simulink model "Progetto_drone_2"  (R2024b)
settings: Solver=VariableStepAuto  StartTime=0.0  StopTime=20  RelTol=1e-3
settings Model: Creator=sugam  LastModifiedBy=3204480343

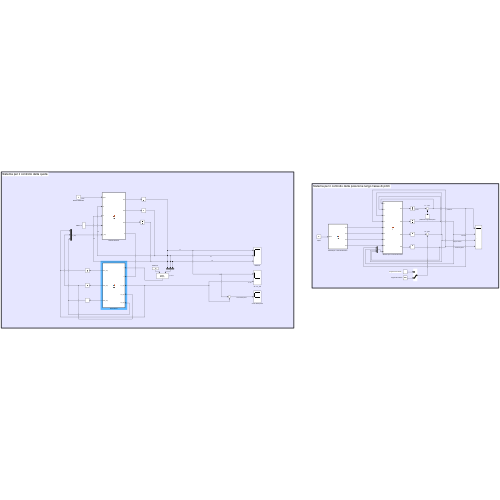
[thumbnail: Simulink's stored preview of the top-level diagram]
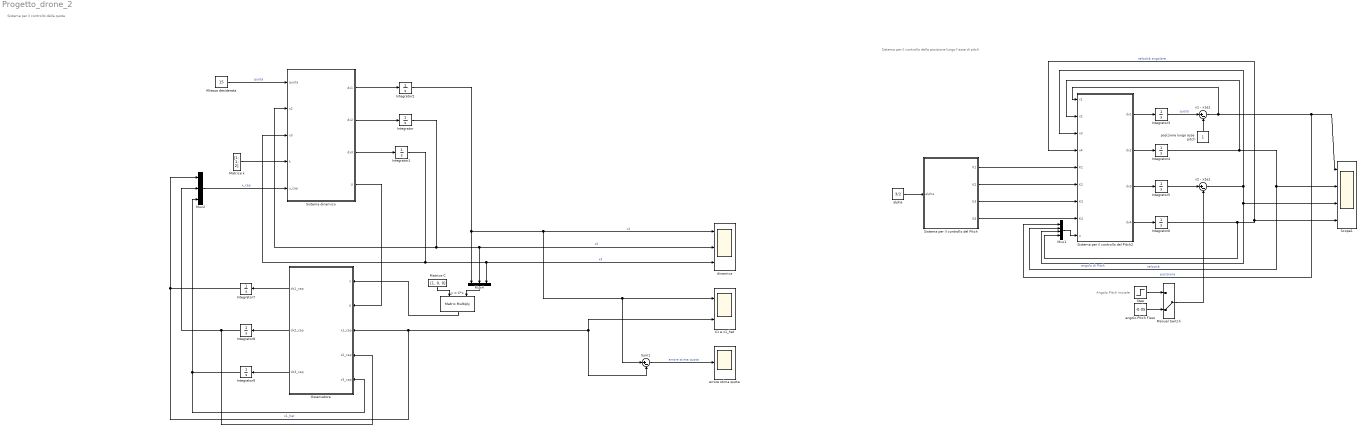
== system Progetto_drone_2 ==
  note: Angolo Pitch iniziale
  note: Sistema per il controllo della quota
  note: Sistema per il controllo della posizione lungo l'asse di pitch
  Altezza desiderata : Constant  Value=15
  Integrator{,1..6} (7 alike) : Integrator
  Integrator7 : Integrator  InitialCondition=2
  Integrator8 : Integrator  InitialCondition=2
  Integrator9 : Integrator  InitialCondition=2
  Manual Switch : ManualSwitch  CurrentSetting=0
  Matrice C : Constant  Value=[1, 0, 0]  VectorParams1D=off
  Matrice k : Constant  Value=[1; 1; 2]  VectorParams1D=off
  Mux1 : Mux
  Mux2 : Mux  Inputs=3
  Mux4 : Mux  Inputs=3
  Osservatore : MATLAB Function  TreatAsAtomicUnit=on
  Scope1 : Scope  NumInputPorts=4
  Sistema dinamico : MATLAB Function  TreatAsAtomicUnit=on
  Sistema per il controllo del Pitch : MATLAB Function  TreatAsAtomicUnit=on
  Sistema per il controllo del Pitch2 : MATLAB Function  TreatAsAtomicUnit=on
  Step : Step  Time=0.01  Before=0.05  After=0  SampleTime=0
  Sum1 : Sum  Inputs=|+-
  X1 e x1_hat : Scope  NumInputPorts=2
  alpha : Constant  Value=3/2
  angolo Pitch Fisso : Constant  Value=-0.05
  dinamica : Scope  NumInputPorts=3
  errore stima quota : Scope
  posizione lungo asse pitch : Constant
  x1 - x1e1 : Sum  Inputs=|+-
  x2 - x2e1 : Sum  Inputs=|+-
  y = C*x : Product  Multiplication=Matrix(*)
  wires:
  alpha/1 -> Sistema per il controllo del Pitch/1(alpha)
  Sistema per il controllo del Pitch/1(K1) -> Sistema per il controllo del Pitch2/5(K1)
  Sistema per il controllo del Pitch/2(K2) -> Sistema per il controllo del Pitch2/6(K2)
  Sistema per il controllo del Pitch/3(K3) -> Sistema per il controllo del Pitch2/7(K3)
  Sistema per il controllo del Pitch/4(K4) -> Sistema per il controllo del Pitch2/8(K4)
  Sistema per il controllo del Pitch2/1(dx1) -> Integrator3/1
  Sistema per il controllo del Pitch2/2(dx2) -> Integrator4/1
  Sistema per il controllo del Pitch2/3(dx3) -> Integrator5/1
  Sistema per il controllo del Pitch2/4(dx4) -> Integrator6/1
  Integrator4/1 -> Sistema per il controllo del Pitch2/2(x2), Scope1/2, Mux1/2  "velocità"
  Integrator6/1 -> Mux1/4, Sistema per il controllo del Pitch2/4(x4), Scope1/4  "velocità angolare"
  Mux1/1 -> Sistema per il controllo del Pitch2/9(u)
  Integrator5/1 -> x2 - x2e1/1
  x2 - x2e1/1 -> Mux1/3, Scope1/3, Sistema per il controllo del Pitch2/3(x3)  "angolo di Pitch"
  Step/1 -> Manual Switch/1
  angolo Pitch Fisso/1 -> Manual Switch/2
  Manual Switch/1 -> x2 - x2e1/2
  posizione lungo asse pitch/1 -> x1 - x1e1/2
  Integrator3/1 -> x1 - x1e1/1  "quota"
  x1 - x1e1/1 -> Sistema per il controllo del Pitch2/1(x1), Mux1/1, Scope1/1  "posizione"
  y = C*x/1 -> Osservatore/1(y)
  Matrice C/1 -> y = C*x/1
  Matrice k/1 -> Sistema dinamico/4(k)
  Mux4/1 -> y = C*x/2
  Mux2/1 -> Sistema dinamico/5(x_cap)  "x_cap"
  Osservatore/2(dx2_cap) -> Integrator8/1
  Osservatore/1(dx1_cap) -> Integrator7/1
  Osservatore/3(dx3_cap) -> Integrator9/1
  Sistema dinamico/3(dx3) -> Integrator1/1
  Integrator7/1 -> X1 e x1_hat/2, Sum1/2, Osservatore/3(x1_cap), Mux2/1  "x1_hat"
  Integrator/1 -> Mux4/2, dinamica/2, Sistema dinamico/2(x2)  "x2"
  Sistema dinamico/1(dx1) -> Integrator2/1
  Sum1/1 -> errore stima quota/1  "errore stima quota"
  Integrator2/1 -> Mux4/1, Sum1/1, X1 e x1_hat/1, dinamica/1  "x1"
  Integrator8/1 -> Osservatore/4(x2_cap), Mux2/2
  Sistema dinamico/2(dx2) -> Integrator/1
  Altezza desiderata/1 -> Sistema dinamico/1(quota)  "quota"
  Integrator1/1 -> Mux4/3, dinamica/3, Sistema dinamico/3(x3)  "x3"
  Integrator9/1 -> Mux2/3, Osservatore/5(x3_cap)
  Sistema dinamico/4(U) -> Osservatore/2(U)

== matlab function Progetto_drone_2/Sistema per il controllo del Pitch2 ==
  data: x1 input; x2 input; x3 input; x4 input; K1 input; K2 input; K3 input; K4 input; u input; dx1 output; dx2 output; dx3 output; dx4 output
function [dx1, dx2, dx3, dx4] = fcn(x1, x2, x3, x4, K1, K2, K3, K4, u)
%Inizializzazione dei parametri inerenti il drone e l'ambiente
g = 9.81;           %forza di gravità che agisce sul drone
I = (1/10)*eye(1);         % momento di inerzia -> valore consiglito 0.02 Kg*m^2
P = 1;              % P parametro che converte l'ingresso 'u' in una coppia per i motori -> valore consigliato 3*10^-7 N*m*s^2

%Sistema non lineare per il controllo della quota verticale descritto dalle
%seguenti equazioni differenziali
%dx1 = x2;
%dx2 = (1/m)*(-Tsin(x3) -cx2);
%dx3 = x4;
%dx4 = (P/I)*u2;

%utilizzo un controllo u1 per mantenere il drone su una quota fissa
%u1 = (T/(cos(theta))*m*g ;

%Il controllo che mi permette di stabilizzare il sistema viene calcolato
%tramite backstepping della madonna, 8 pagine de calcoli mortacci tua
u = (I/P)*(K1*u(1) + K2*u(2) + K3*u(3) + K4*u(4));

%Da questo ottengo il sistema linearizzato nell'intorno del punto di
%equilibrio (xe,ue), dove tutti gli elementi sono pari a zero tranne la x1
%che è libera
dx1 = x2;
dx2 = -g*x3;
dx3 = x4;
dx4 = (P/I)*u;

%x1 posizione lungo l'asse del pitch
%x2 velocita longitudinale
%x3 angolo di pitch
%x4 velocita angolare

== matlab function Progetto_drone_2/Sistema dinamico ==
  data: quota input; dx1 output; dx2 output; x2 input; x3 input; k input; dx3 output; x_cap input; U output
function [dx1, dx2, dx3, U] = fcn(quota, x2, x3, k, x_cap)
%Inizializzazione dei parametri inerenti il drone e l'ambiente
g = 9.81;           % forza di gravità che agisce sul drone
tau = 0.1;          % costante di tempo per generare ritardo nel controllo
ka = 0.1;           % coefficiente di proporzionalità tra x3 ed F
m = 1;              % massa del drone

x3e = sqrt(g*m/ka); % circa uguale a 9.9, x3 equlibrio 

ue = x3e;

%Il controllo che mi permette di stabilizzare il sistema viene calcolato
%tramite la legge di feedback dello stato u = -kx
U = -k(1)*(x_cap(1) - quota) - k(2)*x_cap(2) - k(3)*(x_cap(3) - sqrt(g*m/ka)) + ue ; % u_tilde = u - ue

%Sistema non lineare per il controllo della quota verticale descritto dalle
%seguenti equazioni differenziali
dx1 = x2;
dx2 = (ka/m)*x3^2 - g;
dx3 = (U - x3)/tau;

% x1 quota
% x2 velocità 
% x3 cinematica motore (spinta motore)

== matlab function Progetto_drone_2/Sistema per il controllo del Pitch ==
  data: alpha input; K1 output; K2 output; K3 output; K4 output
function [K1, K2, K3, K4] = fcn(alpha)
%inizializzazione parametri
g = 9.81;

%calcolo delle varie K che fanno parte del controllo come
%u = (I/P)*(K1*x1 + K2*x2 + K3*x3 + K4*x4)
K1 = -(2*(alpha^4) + (6*(alpha^3)) + (-4*(alpha^2)) + (-16*alpha) + (-alpha*(g^2)) -8)/g;
K2 = -(-4*alpha + (-alpha*(g^2)) -4 - (g^2))/g;
K3 = -(3*alpha + 5 + g^2);
K4 = - (3+alpha) ;

== matlab function Progetto_drone_2/Osservatore ==
  data: y input; U input; x1_cap input; x2_cap input; x3_cap input; dx1_cap output; dx2_cap output; dx3_cap output
function [dx1_cap, dx2_cap, dx3_cap] = fcn(y, U, x1_cap, x2_cap, x3_cap)
%Inizializzazione dei parametri inerenti il drone e l'ambiente
g = 9.81;           % forza di gravità che agisce sul drone
tau = 0.1;          % costante di tempo per generare ritardo nel controllo
ka = 0.1;           % coefficiente di proporzionalità tra x3 ed F
m = 1;              % massa del drone

C = [1 0 0];        % Matrice C d'uscita

%valori scelti tali che p(s) è Hurwitz

%le c devono essere tali che il polinomio p(s) = s^3 + c2s^2 + c1s + c0 e
%di Hurwitz: infatti scrivendo su matlab
% p = [1 3 3 1];
% roots_p = roots(p);
% isHurwitz = all(real(roots_p) < 0) %questa variabile deve uscire true (1)


c2 = 3;
c1 = 3;
c0 = 1;

y_cap = C*[x1_cap; x2_cap; x3_cap];

K = 1; % valore scelto empiricamente 

%Sistema non lineare per il controllo della quota verticale descritto dalle
%seguenti equazioni differenziali
dx1_cap = x2_cap + K*c2*(y - y_cap);
dx2_cap = (ka/m)*x3_cap^2 - g + (K^2)*c1*(y - y_cap);
dx3_cap = (U - x3_cap)/tau + (K^3)*c0*(y - y_cap);
